simulink model "suspmod"  (R2023a)
settings: Solver=VariableStepAuto  StartTime=0.0  StopTime=20  MaxStep=0.01  RelTol=1e-3
model workspace (MAT data in the model file):
  M1 = 2500
  M2 = 320
  b1 = 350
  b2 = 15020
  k1 = 80000
  k2 = 500000
libraries: slpidlib x1
settings Model: Creator=guess  LastModifiedBy=guess
settings SolverCC: MaxConsecutiveMinStep=5

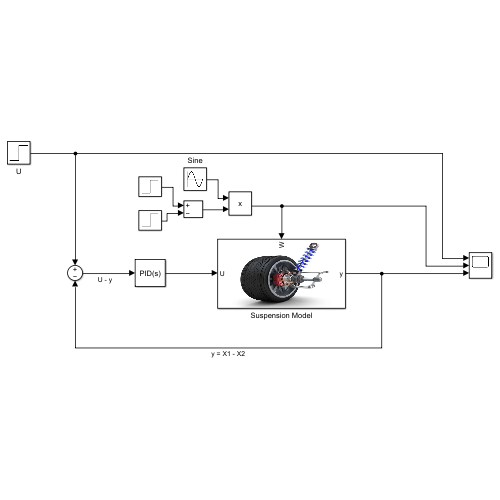
[thumbnail: Simulink's stored preview of the top-level diagram]
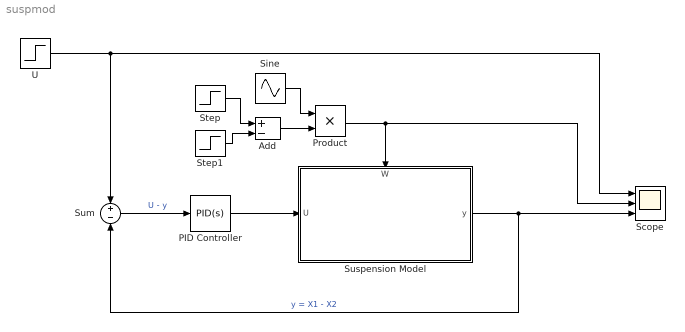
== system suspmod ==
  Add : Sum  Inputs=+-
  PID Controller : slpidlib/PID Controller  Controller=PID  Form=Parallel  TimeDomain=Continuous-time  UseExternalTs=off  SampleTime=-1  IntegratorMethod=Forward Euler  FilterMethod=Forward Euler  ControllerParametersSource=internal  P=10255095.7637267  I=69609208.0107218  UseKiTs=off  D=306794.408293066  N=123710.397061165  UseFilter=on  TunerSelectOption=Transfer Function Based (PID Tuner App)  InitialConditionSource=internal  InitialConditionForIntegrator=0  InitialConditionForFilter=0  DifferentiatorICPrevScaledInput=0  ExternalReset=none  TrackingMode=off  Kt=1  LimitOutput=off  SatLimitsSource=internal  UpperSaturationLimit=inf  LowerSaturationLimit=-inf  LinearizeAsGain=on  AntiWindupMode=none  Kb=1  LimitIntegrator=off  UpperIntegratorSaturationLimit=inf  LowerIntegratorSaturationLimit=-inf  POutMin=[]  POutMax=[]  IOutMin=[]  IOutMax=[]  DOutMin=[]  DOutMax=[]  NOutMin=[]  NOutMax=[]  SumOutMin=[]  SumOutMax=[]  SaturationOutMin=[]  SaturationOutMax=[]  PParamMin=[]  PParamMax=[]  IParamMin=[]  IParamMax=[]  DParamMin=[]  DParamMax=[]  NParamMin=[]  NParamMax=[]  KbParamMin=[]  KbParamMax=[]  KtParamMin=[]  KtParamMax=[]  KbOutMin=[]  KbOutMax=[]  KtOutMin=[]  KtOutMax=[]  IntegratorOutMin=[]  IntegratorOutMax=[]  FilterOutMin=[]  FilterOutMax=[]  SumI1OutMin=[]  SumI1OutMax=[]  SumI2OutMin=[]  SumI2OutMax=[]  SumI3OutMin=[]  SumI3OutMax=[]  SumI4OutMin=[]  SumI4OutMax=[]  SumDOutMin=[]  SumDOutMax=[]  DifferentiatorOutMin=[]  DifferentiatorOutMax=[]  FilterDiffOutCoefMin=[]  FilterDiffOutCoefMax=[]  ReciprocalOutMin=[]  ReciprocalOutMax=[]  SumDenOutMin=[]  SumDenOutMax=[]  SumNumOutMin=[]  SumNumOutMax=[]  DivideOutMin=[]  DivideOutMax=[]  UdiffTsProdOutMin=[]  UdiffTsProdOutMax=[]  NTsProdOutMin=[]  NTsProdOutMax=[]  UintegralTsProdOutMin=[]  UintegralTsProdOutMax=[]  UngainTsProdOutMin=[]  UngainTsProdOutMax=[]  ClampingZeroOutDataTypeStr=Inherit: Inherit via back propagation  ClampingZeroOutMin=[]  ClampingZeroOutMax=[]  FilterDenConstantOutDataTypeStr=Inherit: Inherit via back propagation  FilterDenConstantOutMin=[]  FilterDenConstantOutMax=[]  PCopyOutDataTypeStr=Inherit: Inherit via back propagation  PCopyOutMin=[]  PCopyOutMax=[]  NCopyOutDataTypeStr=Inherit: Inherit via back propagation  NCopyOutMin=[]  NCopyOutMax=[]  IntegratorContinuousStateAttributes=''  IntegratorStateMustResolveToSignalObject=off  IntegratorRTWStateStorageClass=Auto  FilterContinuousStateAttributes=''  FilterStateMustResolveToSignalObject=off  FilterRTWStateStorageClass=Auto  ParallelPVariant=InternalParameters  IdealPVariant=Disabled  IVariant=InternalParameters  DVariant=InternalParameters  IntegratorVariant=Continuous  SatVariant=Disabled  AWVariant=Passthrough  PCopyVariant=Disabled  TRVariant=Disabled  FdbkBlocksVariant=Forward  IdealPFdbkVariant=Disabled  SatFdbkVariant=Disabled  DerivativeFilterVariant=ContFilter  NVariant=InternalParameters  NCopyVariant=Disabled  FilterICVariant=InternalICsFilter  IntegratorICVariant=InternalICs  ExternalResetVariant=Disabled  TRSumVariant=Passthrough  SumFdbkVariant=Disabled  SumVariant=Sum_PID  TsampFilterVariant=InternalTs  TsampNgainVariant=Passthrough  TsampIntegralVariant=Disabled_SignalSpec  ExternalSaturationOutDataTypeStr=Inherit: Same as second input
  Product : Product
  Scope : Scope  NumInputPorts=3
  Sine : Sin  Amplitude=1.5  Frequency=pi/2  Phase=-pi/2  SampleTime=0
  Step : Step  Time=9  SampleTime=0
  Step1 : Step  Time=11  SampleTime=0
  Sum : Sum  Inputs=+-
  Suspension Model : Subsystem
      settings: PortSchema="{\"entries\":[{\"content\":{\"sides\":[{\"content\":{\"connectorIds\":[\"In1\"]},\"type\":\"ConnectorPlacement.EquallySpacedRectSide\",\"uuid\":\"0c28c1ec-f9ef-40c2-897a-1cd7f0d0a3f8\"},{\"content\":{\"connectorIds\":[\"Out1\"],\"side\":\"RIGHT\"},\"type\":\"ConnectorPlacement.EquallySpacedRectSide\",\"uuid\":\"f66e1639-0b60-4b0e-85c7-79f422b8e41d\"},{\"content\":{\"connectorIds\":[\"In2\"],\"side\":\"TOP\"},\"type\":\"ConnectorPlacement.EquallySpacedRectSide\",\"uuid\":\"37b1a9a2-247a-477e-a3e7-940adda032a5\"}]},\"type\":\"ConnectorPlacement.EquallySpacedConnector\",\"uuid\":\"7badcb1b-42f3-4e9e-b526-b8a1f1d68e35\"}],\"packageUris\":[\"http://schema.mathworks.com/mf0/Connector/R2020b\"],\"version\":\"1.0\"}"
      mask Display: image('Suspension.png'); % Use "Edit Image" on toolstrip to change.
  U : Step  SampleTime=0
  wires:
  Suspension Model/1(y) -> Sum/2, Scope/3  "y = X1 - X2"
  PID Controller/1 -> Suspension Model/1(U)
  U/1 -> Sum/1, Scope/1
  Sum/1 -> PID Controller/1  "U - y"
  Product/1 -> Scope/2, Suspension Model/2(W)
  Step/1 -> Add/1
  Step1/1 -> Add/2
  Add/1 -> Product/2
  Sine/1 -> Product/1

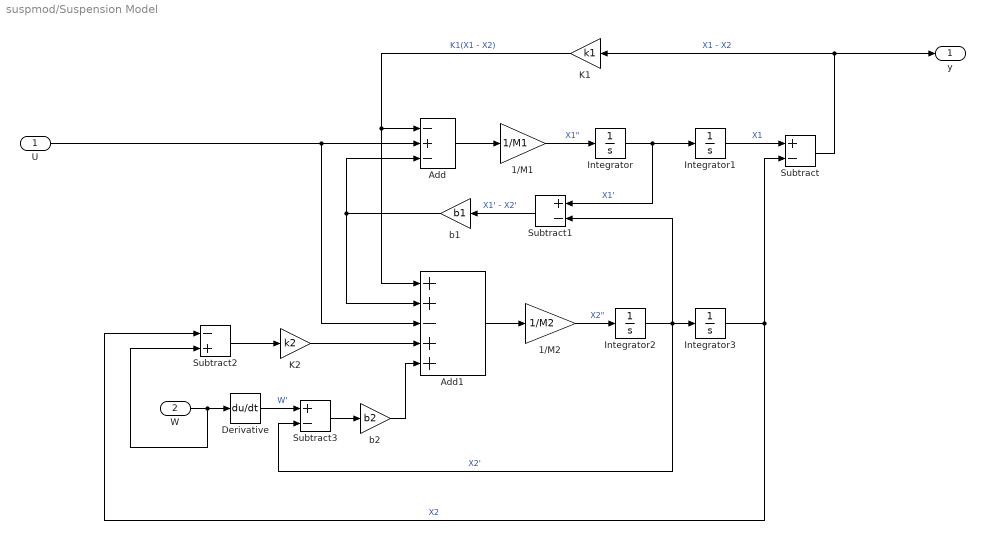
== system suspmod/Suspension Model ==
  U : Inport
  W : Inport  Port=2
  1/M1 : Gain  Gain=1/M1
  1/M2 : Gain  Gain=1/M2
  Add : Sum  Inputs=-+-
  Add1 : Sum  Inputs=++-++
  Derivative : Derivative
  Integrator{,1..3} (4 alike) : Integrator
  K1 : Gain  Gain=k1
  K2 : Gain  Gain=k2
  Subtract : Sum  Inputs=+-
  Subtract1 : Sum  Inputs=+-
  Subtract2 : Sum  Inputs=-+
  Subtract3 : Sum  Inputs=+-
  b1 : Gain  Gain=b1
  b2 : Gain  Gain=b2
  y : Outport
  wires:
  Integrator2/1 -> Subtract1/2, Integrator3/1, Subtract3/2  "X2'"
  Integrator/1 -> Subtract1/1, Integrator1/1  "X1'"
  Subtract2/1 -> K2/1
  Derivative/1 -> Subtract3/1  "W'"
  Integrator3/1 -> Subtract/2, Subtract2/1  "X2"
  1/M2/1 -> Integrator2/1  "X2\""
  b1/1 -> Add1/2, Add/3
  Integrator1/1 -> Subtract/1  "X1"
  W/1 -> Derivative/1, Subtract2/2
  K1/1 -> Add/1, Add1/1  "K1(X1 - X2)"
  Subtract/1 -> y/1, K1/1  "X1 - X2"
  Subtract1/1 -> b1/1  "X1' - X2'"
  Add/1 -> 1/M1/1
  Add1/1 -> 1/M2/1
  1/M1/1 -> Integrator/1  "X1\""
  U/1 -> Add/2, Add1/3
  K2/1 -> Add1/4
  Subtract3/1 -> b2/1
  b2/1 -> Add1/5
